simulink library "rtlsdr_book_library"  (R2018a)
settings: Solver=ode45  StartTime=0.0  StopTime=10.0  RelTol=1e-3  EnableMultiTasking=on
undefined symbols (not defined in the file): costas, den, dfilt, fdesignblkfcn, frm, gcbh, iir, num, rtlsdr_frmsize, rtlsdr_fs, src
libraries: dspsigops x6, commsynccomp2 x4, dspsrcs4 x2, dspstat3 x2, dspobslib x2, simulink_extras x2, dspmtrx3 x2, dsparch4 x1, $bdroot x1, dspspect3 x1, commrflib2 x1
(part 2 of 5)

== system rtlsdr_book_library/Additional Tools/Model Information ==
  Model Information : Subsystem
      mask help:
      | html = [html,'</br></br>',...
      |                '<table style="width:100%">',...
      |                '<tr>',...
      |                     '<td align="center" rowspan=2>',...  COL1 ROW 1
      |                         '<a href="matlab:openpdfnameddest_slxfile" STYLE="text-decoration: none">',...
      |                         '<img src="',imagepath_book,'" title="Click here to open the book at the corresponding exercise"  align="middle"/></a>',...
      |                     '</td>'];
      |         if file.videourl ~= ''''
      |             html = [html,...
      |                     '<td align="center">',...  COL 2 ROW 1
      |                         '<a href="',file.videourl,'" STYLE="text-decoration: none">',...
      |                         '<img src="',imagepath_video,'" title="Click here to watch the video"  align="middle"/></a>',...
      |                     '</td>'];
      |         end
      |         html = [html,'</tr>'];
      |
      |         if file.videourl ~= ''''
      |             html = [html,...
      |                 '<tr>',...
      |                     '<td align="center">',... COL 2 ROW 2
      |                         '<a href="',file.videourl,'" STYLE="text-decoration: none; color: #007193">',...
      |                         '<h4></br>Click here to watch the video</h4></a>',...
      |                     '</td>',...
      |                 '</tr>'];
      |         else
      |             html = [html,... ROW 2
      |                 '<tr></tr>'];
      |         end
      |         html = [html,...
      |                 '<tr>',...
      |                     '<td align="center" rowspan="2">',... COL 1 ROW 3
      |                         '<a href="matlab:openpdfnameddest_slxfile" STYLE="text-decoration: none; color: #007193">',...
      |                         '<h4></br>Click here to open the book</br>at the corresponding exercise</h4></a>',...
      |                     '</td>',...
      |                 '</tr>'];
      mask DialogControl DescGroupVar Prompt: Model Information
      mask Display:
      | % if java is installed and the help browser can be launched
      | if usejava('swing')
      | 
      |     % try to pull model properties into block
      |     try
      | 
      |         %% IMPORT FILE PARAMS
      | 
      |         % find rtlsdr book root folder
      |         root = which('rtlsdr_book_library');
      |         root = root(1:end-length('rtlsdr_book_library/rtlsdr_book_library.slx'));
      | 
      |         % find filename, path etc
      |         file.path = which(bdroot);
      |         [parentfolder,filenamenoext,fileext] = fileparts(file.path);
      |         file.relativepath = ['...',file.path(length(root):end)];
      |         file.name =[filenamenoext,fileext];
      | 
      |         % load file information cell array
      |         load('fileinfo.mat');
      | 
      |         % search to find file information
      |         row = find(ismember(fileinfo,file.name));
      | 
      |         % get remaining file information
      |         file.title = char(fileinfo(row,2));
      |         file.author = char(fileinfo(row,3));
      |         file.date = char(fileinfo(row,4));
      |         file.pdfnameddest = char(fileinfo(row,5));
      |         file.videourl = char(fileinfo(row,6));
      |         file.info1 = char(fileinfo(row,7));
      |         file.info2 = char(fileinfo(row,8));
      |         file.infoi = char(fileinfo(row,9));
      | 
      |         %% CHECK BLOCK POSITION
      |         blkpos = get_param(gcb,'Position');
      |         set_param(gcb,'Position',[blkpos(1),blkpos(2),blkpos(3),blkpos(2)+150]);
      | 
      |         %% BLOCK TEXT TITLE
      |         blktitlelen = blkpos(3)-blkpos(1)-450;
      |         blktitlecharlen = round(blktitlelen/11);
      |         blktitle = file.title;
      |         % check if title is too long to fit on one line
      |         if length(blktitle) > blktitlecharlen
      |             % find out where spaces are
      |             titlespaces = isspace(blktitle);
      |             for i = blktitlecharlen:-1:1
      |                 % if there is a space at position i
      |                 if titlespaces(i)==1
      |                     % replace with new line char
      |                     blktitle(i)=char(10);
      |                     blktitlebreakpos = i;
      |                     % break loop
      |                     break;
      |                 end
      |             end
      |         end
      |         % check if title is too long to fit on two lines
      |         if length(blktitle) > 2*blktitlecharlen
      |             % find out where spaces are
      |             titlespaces = isspace(blktitle);
      |             for i = 2*blktitlecharlen:-1:blktitlecharlen
      |                 % if there is a space at position i
      |                 if titlespaces(i)==1
      |                     % replace with new line char
      |                     blktitle(i)=char(10);
      |                     % break loop
      |                     break;
      |                 end
      |             end
      |         end
      |         % format string for mask display
      |         blkmsg = ['\bf\fontsize{20}',blktitle,'\fontsize{22}',char(10),...
      |                   '\rm\fontsize{16}www.desktopSDR.com\fontsize{18}',char(10),...
      |                   '\rm\fontsize{14}Double click for more information'];
      | 
      | 
      |         %% CREATE PARAMS FOR HTML
      |         % get MATLAB version
      |         MATLABversion = num2str(get_param(gcs,'Version'));
      |         if MATLABversion(1:3)=='8.2'
      |             file.MATLABversion = ['Last saved in Simulink version ',MATLABversion(1:3),' – R2013b'];
      |         elseif MATLABversion(1:3)=='8.3'
      |             file.MATLABversion = ['Last saved in Simulink version ',MATLABversion(1:3),' – R2014a'];
      |         elseif MATLABversion(1:3)=='8.4'
      |             file.MATLABversion = ['Last saved in Simulink version ',MATLABversion(1:3),' – R2014b'];
      |         elseif MATLABversion(1:3)=='8.5'
      |             file.MATLABversion = ['Last saved in Simulink version ',MATLABversion(1:3),' – R2015a'];
      |         elseif MATLABversion(1:3)=='8.6'
      |             file.MATLABversion = ['Last saved in Simulink version ',MATLABversion(1:3),' – R2015b'];
      |         else
      |             file.MATLABversion = ['Last saved in Simulink version ',MATLABversion(1:3)];
      |         end
      |         % image hyperlinks
      |         imagepath_book = [root,'rtlsdr_book_library/block_icons/icon__book.png'];
      |         imagepath_desktopSDR = [root,'rtlsdr_book_library/block_icons/icon__desktopSDR.png'];
      |         imagepath_video = [root,'rtlsdr_book_library/block_icons/icon__video.png'];
      | 
      | 
      |         %% CREATE HTML WEBPAGE FOR OPEN FUNCTION CALLBACK
      |         % create table at the top
      |         html = ['text://<html>',...
      |                 '<title>',bdroot,' - ',file.title,'</title>',...
      |                 '<body>',...
      |                 '<table style="width:100%" border=0 cellspacing=0 cellpadding=20">',...
      |                     '<tr>',...
      |                         '<td bgcolor="#007193" style="width: 100%;">',...
      |                         '<center><a href=http://www.desktopSDR.com>',...
      |                             '<img src="',imagepath_desktopSDR,'" title="Go to desktopSDR.com"  align="middle"/>',...
      |                         '</a></center>',...
      |                         '</td>',...
      |                     '</tr>',...
      |                 '</table></br></br>',...
      |                 '<table style="width:100%">',...
      |                     '<tr>',...
      |                         '<td class="expand"><font color="#323232" face="verdana"><h2>Model Title:</h2></td>',...
      |                         '<td><font color="#323232" face="verdana"><h2>',file.title,'</h2></td>',...
      |                     '</tr>',...
      |                     '<tr>'...
      |                         '<td class="expand"><font color="#323232" face="verdana"><h3>Model Filepath:</h3></td>',...
      |                         '<td><font color="#323232" face="verdana"><h3>',file.relativepath,'</h3></td>',...
      |                     '</tr>'...
      |                     '<tr>'...
      |                         '<td class="expand"><font color="#323232" face="verdana"><h5>Model Author:</h5></td>',...
      |                         '<td><font color="#323232" face="verdana"><h5>',file.author,'</h5></td>',...
      |                     '</tr>'...
      |                     '<tr>'...
      |                         '<td class="expand"><font color="#323232" face="verdana"><h5>Model Date:</h5></td>',...
      |                         '<td><font color="#323232" face="verdana"><h5>',file.date,'</h5></td>',...
      |                     '</tr>'...
      |                     '<tr>'...
      |                         '<td class="expand"><font color="#323232" face="verdana"><h5>Simulink Version:</h5></td>',...
      |                         '<td><font color="#323232" face="verdana"><h5>',file.MATLABversion,'</h5></td>',...
      |                     '</tr>'...
      |                     '<tr>'...
      |                         '<td><font color="#323232" face="verdana"><h5>Exercise introduction:</h5></td>',...
      |                     '</tr>'...
      |                 '</table>'];
      |         % add info paragraphs if they are populated
      |         if file.info1 ~= ''''
      |             html = [html,'<font color="#757575" face="verdana"><p align="justify">',file.info1,'</p>'];
      |         end
      |         if file.info2 ~= ''''
      |             html = [html,'<font color="#757575" face="verdana"><p align="justify">',file.info2,'</p>'];
      |         end
      |         if file.infoi ~= ''''
      |             html = [html,'<p align="justify"><i>',file.infoi,'</i></p>'];
      |         end
      |         % add hyperlinks in second table (book only if no video is provided)
      |         html = [html,'</br></br>',...
      |                '<table style="width:100%">',...
      |                '<tr>',...
      |                     '<td align="center">',...  COL 1 ROW 1
      |                         '<a href="matlab:openpdfnameddest_slxfile" STYLE="text-decoration: none">',...
      |                         '<img src="',imagepath_book,'" title="Click here to open the book at the corresponding exercise"  align="middle"/></a>',...
      |                     '</td>'];
      |         if file.videourl ~= ''''
      |             html = [html,...
      |                     '<td align="center">',...  COL 2 ROW 1
      |                         '<a href="',file.videourl,'" STYLE="text-decoration: none">',...
      |                         '<img src="',imagepath_video,'" title="Click here to watch the video"  align="middle"/></a>',...
      |                     '</td>'];
      |         end
      |         html = [html,'</tr>'];
      | 
      |         html = [html,...
      |                 '<tr>',...
      |                     '<td align="center" rowspan="2">',... COL 1 ROW 2
      |                         '<a href="matlab:openpdfnameddest_slxfile" STYLE="text-decoration: none; color: #007193">',...
      |                         '<h4></br>Click here to open the book</br>at the corresponding exercise</h4></a>',...
      |                     '</td>'];
      |         if file.videourl ~= ''''
      |             html = [html,...
      |                     '<td align="center">',... COL 2 ROW 2
      |                         '<a href="',file.videourl,'" STYLE="text-decoration: none; color: #007193">',...
      |                         '<h4></br>Click here to watch the video</h4></a>',...
      |                     '</td>',...
      |                 '</tr>'];
      |         else
      |             html = [html,... ROW 2
      |                 '</tr>'];
      |         end
      | 
      |         % finish table
      |         html = [html,'</table>'];
      | 
      |         % legal information
      |         html = [html,...
      |                 '<font color="#757575" face="verdana" size=1></br></br></br></br></br></br>',...
      |                 '</br><strong>Software, Simulation Examples and Design Exercises Licence Agreement</strong>',...
      |                 '</br><p align="justify">This license agreement refers to the simulation examples, design exercises and files, and associated software MATLAB and Simulink resources that accompany the book:',...
      |                 '</br></br>&nbsp;&nbsp;&nbsp;<em>Title: Software Defined Radio using MATLAB & Simulink and the RTL-SDR',...
      |                 '</br>&nbsp;&nbsp;&nbsp;Published by Strathclyde Academic Media, 2015',...
      |                 '</br>&nbsp;&nbsp;&nbsp;Authored by Robert W. Stewart, Kenneth W. Barlee, Dale S.W. Atkinson, and Louise H. Crockett</em>',...
      |                 '</br></br><p align="justify">and made available as a download from <a href="http://www.desktopSDR.com" STYLE="text-decoration: none">www.desktopSDR.com</a> or variously acquired by other means such as via USB storage, cloud storage, disk or any other electronic or optical or magnetic storage mechanism. These files and associated software may be used subject to the terms of agreement of the conditions below:',...
      |                 '</br></br>&nbsp;&nbsp;&nbsp;<em>Copyright © 2015 Robert W. Stewart, Kenneth W. Barlee, Dale S.W. Atkinson, and Louise H. Crockett. All rights reserved.</em>',...
      |                 '</br></br><p align="justify">Redistribution and use in source and binary forms, with or without modification, are permitted provided that the following conditions are met:',...
      |                 '<ol type="1">',...
      |                 '</br><li>Redistributions of source code must retain the above copyright notice, this list of conditions and the following disclaimer.</li>',...
      |                 '</br><li>Redistributions in binary form must reproduce the above copyright notice, this list of conditions and the following disclaimer in the documentation and/or other materials provided with the distribution.</li>',...
      |                 '</br><li>Neither the name of the copyright holder nor the names of its contributors may be used to endorse or promote products derived from this software without specific prior written permission.</li>',...
      |                 '</br><li>In all cases, the software is, and all modifications and derivatives of the software shall be, licensed to you solely for use in conjunction with The MathWorks, Inc. products and service offerings.</li>',...
      |                 '</ol>',...
      |                 '</br><p align="justify">THIS SOFTWARE IS PROVIDED BY THE COPYRIGHT HOLDERS AND CONTRIBUTORS "AS IS" AND ANY EXPRESS OR IMPLIED WARRANTIES, INCLUDING, BUT NOT LIMITED TO, THE IMPLIED WARRANTIES OF MERCHANTABILITY AND FITNESS FOR A PARTICULAR PURPOSE ARE DISCLAIMED. IN NO EVENT SHALL THE COPYRIGHT HOLDER OR CONTRIBUTORS BE LIABLE FOR ANY DIRECT, INDIRECT, INCIDENTAL, SPECIAL, EXEMPLARY, OR CONSEQUENTIAL DAMAGES (INCLUDING, BUT NOT LIMITED TO, PROCUREMENT OF SUBSTITUTE GOODS OR SERVICES; LOSS OF USE, DATA, OR PROFITS; OR BUSINESS INTERRUPTION) HOWEVER CAUSED AND ON ANY THEORY OF LIABILITY, WHETHER IN CONTRACT, STRICT LIABILITY, OR TORT (INCLUDING NEGLIGENCE OR OTHERWISE) ARISING IN ANY WAY OUT OF THE USE OF THIS SOFTWARE, EVEN IF ADVISED OF THE POSSIBILITY OF SUCH DAMAGE.</p>',...
      |                 '</br><strong>Audio Tracks used in Simulations Examples and Design Exercises</strong>',...
      |                 '<p align="justify">The music and vocal files used within the Examples files and software within the book were variously written, arranged, performed, recorded and produced by Garrey Rice, Adam Struth, Jamie Struth, Iain Thistlethwaite and also Marshall Craigmyle who collectively, and individually where appropriate, assert and retain all of their copyright, performance and artistic rights. Permission to use and reproduce this music is granted for all purposes associated with MATLAB and Simulink software and the simulation examples and design exercises files that accompany this book. Requests to use the music for any other purpose should be directed to:  info@desktopSDR.com. For information on music track names, full credits, and links to the musicians please refer to <a href="http://www.desktopSDR.com/more/audio" STYLE="text-decoration: none">www.desktopSDR.com/more/audio</a>.</p></br></br>'];
      | 
      |         % finish HTML code
      |         html = [html,...
      |                 '</font></body>',...
      |                 '</html>'];
      | 
      |         % set callback
      |         cb = ['web(''',html,''');'];
      |         set_param(gcb,'OpenFcn',eval('cb'));
      | 
      | 
      |     catch %% CANNOT LOAD PROPERTIES
      | 
      |         % format string for mask display
      |         blkmsg = 'Unable to load model information';
      |         % clear openfcn callback
      |         set_param(gcb,'OpenFcn',' ');
      | 
      |     end
      | end
      | 
      | %% DISPLAY TEXT ON BLOCK
      | text(415,75,blkmsg,'texmode','on','horizontalAlignment','left');
      | 
      | %% DISPLAY IMAGE ON BLOCK
      | try
      |     root = which('rtlsdr_book_library');
      |     root = root(1:end-length('rtlsdr_book_library/rtlsdr_book_library.slx'));
      |     imagepath = [root,'rtlsdr_book_library/block_icons/icon__booklogo.png'];
      |     image(imagepath,[0,0,400,150]);
      | end

== system rtlsdr_book_library/Additional Tools/Remove DC Component ==
  sig_in : Inport
  Mean : dspstat3/Mean  run=off  reset_popup=None  InputProcessing=Columns as channels (frame based)  directionMode=Each column  dimension=1  treatSBRowAsCol=on  roiEnable=off  roiType=Rectangles  roiPortion=Entire ROI  roiOutput=Individual statistics for each ROI  roiFlag=off  outputDataTypeStr=Inherit: Same as accumulator  outputLastDataTypeStr=Inherit: Same as accumulator  outputMin=[]  outputMax=[]  roundingMode=Floor  overflowMode=off
  Subtract : Sum  Inputs=+-
  sig_out : Outport
  wires:
  Subtract/1 -> sig_out/1
  sig_in/1 -> Subtract/1, Mean/1
  Mean/1 -> Subtract/2

== system rtlsdr_book_library/Additional Tools/Save RTL-SDR Data ==
  note: write data in 1D array to timeseries
  data_in : Inport
  Reshape : Reshape
  To File : ToFile  Filename=rtlsdr_data.mat  MatrixName=rtlsdr_data  SaveFormat=Timeseries
  wires:
  data_in/1 -> Reshape/1
  Reshape/1 -> To File/1

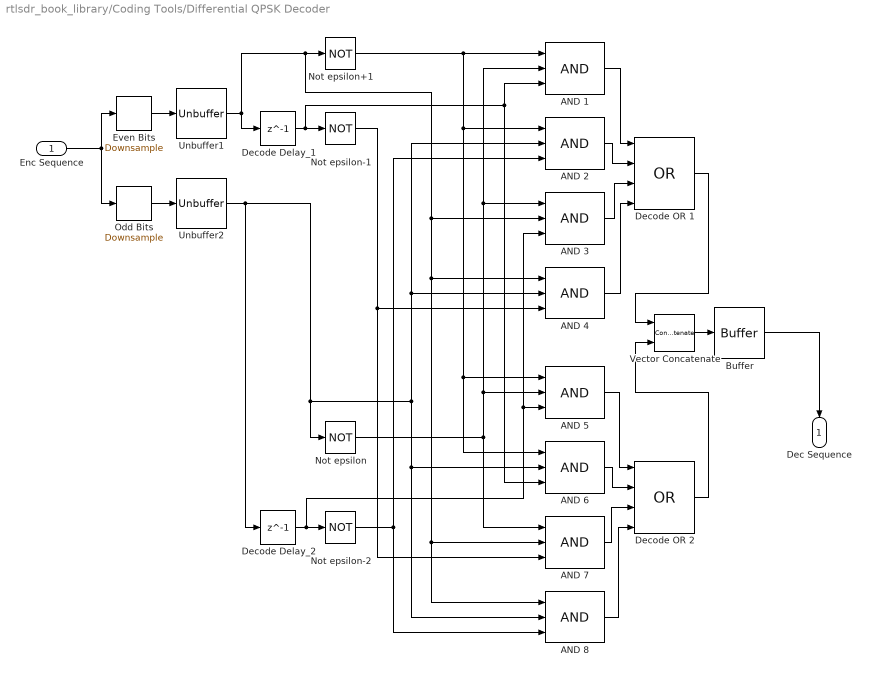
== system rtlsdr_book_library/Coding Tools/Differential QPSK Decoder ==
  Enc Sequence : Inport
  AND {1..8} (8 alike) : Logic  Inputs=3  IconShape=distinctive  AllPortsSameDT=off  OutDataTypeStr=boolean
  Buffer : Buffer  N=op_buff_len
  Decode Delay_1 : Delay  DelayLength=1  InitialCondition=0
  Decode Delay_2 : Delay  DelayLength=1  InitialCondition=0
  Decode OR 1 : Logic  Operator=OR  Inputs=4  IconShape=distinctive  AllPortsSameDT=off  OutDataTypeStr=boolean
  Decode OR 2 : Logic  Operator=OR  Inputs=4  IconShape=distinctive  AllPortsSameDT=off  OutDataTypeStr=boolean
  Even Bits : dspsigops/Downsample  N=2  phase=1  InputProcessing=Columns as channels (frame based)  RateOptions=Enforce single-rate processing  smode=Allow multirate  fmode=Maintain input frame size  ic=0
      settings: SourceProductName=DSP System Toolbox  SourceProductBaseCode=DS
  Not epsilon : Logic  Operator=NOT  Inputs=3  IconShape=distinctive  AllPortsSameDT=off  OutDataTypeStr=boolean
  Not epsilon+1 : Logic  Operator=NOT  Inputs=3  IconShape=distinctive  AllPortsSameDT=off  OutDataTypeStr=boolean
  Not epsilon-1 : Logic  Operator=NOT  Inputs=3  IconShape=distinctive  AllPortsSameDT=off  OutDataTypeStr=boolean
  Not epsilon-2 : Logic  Operator=NOT  Inputs=3  IconShape=distinctive  AllPortsSameDT=off  OutDataTypeStr=boolean
  Odd Bits : dspsigops/Downsample  N=2  phase=0  InputProcessing=Columns as channels (frame based)  RateOptions=Enforce single-rate processing  smode=Allow multirate  fmode=Maintain input frame size  ic=0
      settings: SourceProductName=DSP System Toolbox  SourceProductBaseCode=DS
  Unbuffer1 : Unbuffer
  Unbuffer2 : Unbuffer
  Vector Concatenate : Concatenate
  Dec Sequence : Outport
  wires:
  Not epsilon-2/1 -> AND 2/3, AND 8/3
  Decode OR 2/1 -> Vector Concatenate/2
  Decode Delay_2/1 -> Not epsilon-2/1, AND 3/3, AND 5/3
  Unbuffer1/1 -> Not epsilon+1/1, AND 7/2, AND 8/1, AND 4/1, AND 3/2, Decode Delay_1/1
  Buffer/1 -> Dec Sequence/1
  AND 5/1 -> Decode OR 2/1
  AND 2/1 -> Decode OR 1/2
  Enc Sequence/1 -> Odd Bits/1, Even Bits/1
  AND 3/1 -> Decode OR 1/3
  AND 7/1 -> Decode OR 2/3
  Not epsilon+1/1 -> AND 1/1, AND 6/1, AND 5/1, AND 2/1
  AND 6/1 -> Decode OR 2/2
  Not epsilon/1 -> AND 3/1, AND 1/2, AND 5/2, AND 7/1
  AND 1/1 -> Decode OR 1/1
  AND 4/1 -> Decode OR 1/4
  Even Bits/1 -> Unbuffer1/1
  Odd Bits/1 -> Unbuffer2/1
  Decode OR 1/1 -> Vector Concatenate/1
  Not epsilon-1/1 -> AND 7/3, AND 4/3
  Unbuffer2/1 -> Not epsilon/1, AND 2/2, AND 4/2, AND 6/2, AND 8/2, Decode Delay_2/1
  Decode Delay_1/1 -> Not epsilon-1/1, AND 1/3, AND 6/3
  AND 8/1 -> Decode OR 2/4
  Vector Concatenate/1 -> Buffer/1

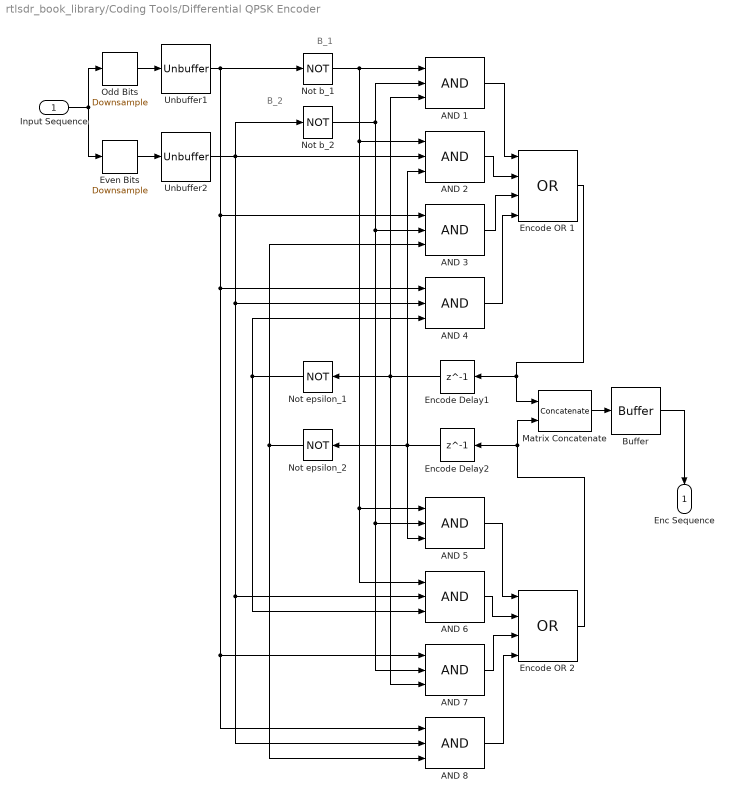
== system rtlsdr_book_library/Coding Tools/Differential QPSK Encoder ==
  note: B_2
  note: B_1
  Input Sequence : Inport
  AND {1..8} (8 alike) : Logic  Inputs=3  IconShape=distinctive  AllPortsSameDT=off  OutDataTypeStr=boolean
  Buffer : Buffer  N=op_buff_len
  Encode Delay1 : Delay  DelayLength=1  InitialCondition=0
  Encode Delay2 : Delay  DelayLength=1  InitialCondition=0
  Encode OR 1 : Logic  Operator=OR  Inputs=4  IconShape=distinctive  AllPortsSameDT=off  OutDataTypeStr=boolean
  Encode OR 2 : Logic  Operator=OR  Inputs=4  IconShape=distinctive  AllPortsSameDT=off  OutDataTypeStr=boolean
  Even Bits : dspsigops/Downsample  N=2  phase=1  InputProcessing=Columns as channels (frame based)  RateOptions=Enforce single-rate processing  smode=Allow multirate  fmode=Maintain input frame size  ic=0
      settings: SourceProductName=DSP System Toolbox  SourceProductBaseCode=DS
  Matrix Concatenate : Concatenate  ConcatenateDimension=2
  Not b_1 : Logic  Operator=NOT  Inputs=3  IconShape=distinctive  AllPortsSameDT=off  OutDataTypeStr=boolean
  Not b_2 : Logic  Operator=NOT  Inputs=3  IconShape=distinctive  AllPortsSameDT=off  OutDataTypeStr=boolean
  Not epsilon_1 : Logic  Operator=NOT  Inputs=3  IconShape=distinctive  AllPortsSameDT=off  OutDataTypeStr=boolean
  Not epsilon_2 : Logic  Operator=NOT  Inputs=3  IconShape=distinctive  AllPortsSameDT=off  OutDataTypeStr=boolean
  Odd Bits : dspsigops/Downsample  N=2  phase=0  InputProcessing=Columns as channels (frame based)  RateOptions=Enforce single-rate processing  smode=Allow multirate  fmode=Maintain input frame size  ic=0
      settings: SourceProductName=DSP System Toolbox  SourceProductBaseCode=DS
  Unbuffer1 : Unbuffer
  Unbuffer2 : Unbuffer
  Enc Sequence : Outport
  wires:
  Encode Delay1/1 -> Not epsilon_1/1, AND 1/3, AND 7/3
  Encode Delay2/1 -> Not epsilon_2/1, AND 5/3, AND 2/3
  Not epsilon_2/1 -> AND 8/3, AND 3/3
  AND 1/1 -> Encode OR 1/1
  AND 8/1 -> Encode OR 2/4
  Even Bits/1 -> Unbuffer2/1
  Input Sequence/1 -> Even Bits/1, Odd Bits/1
  Odd Bits/1 -> Unbuffer1/1
  Encode OR 2/1 -> Matrix Concatenate/2, Encode Delay2/1
  Encode OR 1/1 -> Matrix Concatenate/1, Encode Delay1/1
  AND 2/1 -> Encode OR 1/2
  Not b_2/1 -> AND 7/2, AND 5/2, AND 3/2, AND 1/2
  Unbuffer1/1 -> Not b_1/1, AND 3/1, AND 4/1, AND 7/1, AND 8/1
  AND 6/1 -> Encode OR 2/2
  AND 7/1 -> Encode OR 2/3
  AND 5/1 -> Encode OR 2/1
  Not epsilon_1/1 -> AND 6/3, AND 4/3
  AND 4/1 -> Encode OR 1/4
  Not b_1/1 -> AND 1/1, AND 6/1, AND 5/1, AND 2/1
  AND 3/1 -> Encode OR 1/3
  Unbuffer2/1 -> AND 2/2, AND 4/2, AND 6/2, AND 8/2, Not b_2/1
  Matrix Concatenate/1 -> Buffer/1
  Buffer/1 -> Enc Sequence/1

== system rtlsdr_book_library/Data Comms Sources and Sinks/  ASCII Transfer Binary Source ==
  MATLAB Function : MATLAB Function  TreatAsAtomicUnit=on
  Obtain Frame (header & data) : Constant  Value=src.master_frame  VectorParams1D=off  SampleTime=1/src.fs*(length(src.master_frame))
  Obtain count_lim : Constant  Value=src.count_lim  VectorParams1D=off  SampleTime=1/src.fs*(length(src.master_frame))
  data_out : Outport
  wires:
  Obtain count_lim/1 -> MATLAB Function/1(count_lim)
  Obtain Frame (header & data)/1 -> MATLAB Function/2(master_frame)
  MATLAB Function/1(frame_output) -> data_out/1

== system rtlsdr_book_library/Data Comms Sources and Sinks/ASCII Decoding ==
  frame_payload_in : Inport
  Ascii Length : Constant  Value=ascii_len  VectorParams1D=off  OutDataTypeStr=single  FramePeriod=4096/240e3
  Binary to ASCII : MATLAB Function  TreatAsAtomicUnit=on
      mask init:
      | %% FIGURE SETUP        
      | %figure;
      | 
      | % resize
      | %window_x = 500;
      | %window_y = 500;
      | %window_width = 500;
      | %window_height = 110;
      | %set(gcf, 'Position', [window_x window_y window_width window_height]);
      | %set(gcf, 'menubar', 'none');
  Message Length : Constant  Value=msg_len  VectorParams1D=off  OutDataTypeStr=single  FramePeriod=-1
  wires:
  Message Length/1 -> Binary to ASCII/2(msg_len)
  Ascii Length/1 -> Binary to ASCII/3(ascii_len)
  frame_payload_in/1 -> Binary to ASCII/1(msg)

== system rtlsdr_book_library/Data Comms Sources and Sinks/Image Reconstruction ==
  frame_in : Inport
  Binary Length of Pixel : Constant  Value=frm.binary_len  VectorParams1D=off  OutDataTypeStr=single  FramePeriod=-1
  Image Reconstruction : MATLAB Function  TreatAsAtomicUnit=on
  wires:
  frame_in/1 -> Image Reconstruction/1(frame_in)
  Binary Length of Pixel/1 -> Image Reconstruction/2(binary_len)

== system rtlsdr_book_library/Data Comms Sources and Sinks/Image Transfer Binary Source ==
  MATLAB Function : MATLAB Function  TreatAsAtomicUnit=on
  Obtain Frame (header & data) : Constant  Value=frm.master_frame  VectorParams1D=off  SampleTime=1/frm.fs*(frm.frame_len)
  Obtain number of frames : Constant  Value=frm.no_of_frames  VectorParams1D=off  SampleTime=1/frm.fs*(frm.frame_len)
  data_out : Outport
  wires:
  Obtain number of frames/1 -> MATLAB Function/1(count_lim)
  Obtain Frame (header & data)/1 -> MATLAB Function/2(master_frame)
  MATLAB Function/1(frame_output) -> data_out/1

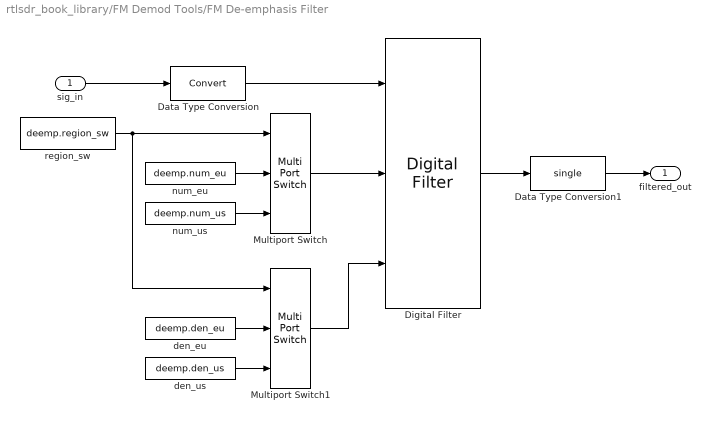
== system rtlsdr_book_library/FM Demod Tools/FM De-emphasis Filter ==
  sig_in : Inport
  Data Type Conversion : DataTypeConversion
  Data Type Conversion1 : DataTypeConversion  OutDataTypeStr=single
  Digital Filter : dspobslib/Digital Filter  TypePopup=IIR (poles & zeros)  IIRFiltStruct=Direct form I  AllPoleFiltStruct=Direct form  FIRFiltStruct=Direct form  CoeffSource=Input port(s)  NumCoeffs=[1 2]  DenCoeffs=[1 0.1]  BiQuadCoeffs=[1 0.3 0.4 1 0.1 0.2]  LatticeCoeffs=[0.2 0.4]  denIgnore=off  FiltPerSampPopup=One filter per frame  IC=0  ICnum=0  ICden=0  roundingMode=Floor  overflowMode=off  ScaleValues=1  scaleValueFracLength=14  stageInFracLength=15  stageOutFracLength=15  FilterSource=Input port(s)  dfiltObjectName=dfilt.df1(num,den)  InputProcessing=Columns as channels (frame based)
      settings: SourceProductName=DSP System Toolbox  SourceProductBaseCode=DS
  Multiport Switch : MultiPortSwitch  Inputs=2
  Multiport Switch1 : MultiPortSwitch  Inputs=2
  den_eu : Constant  Value=deemp.den_eu
  den_us : Constant  Value=deemp.den_us
  num_eu : Constant  Value=deemp.num_eu
  num_us : Constant  Value=deemp.num_us
  region_sw : Constant  Value=deemp.region_sw
  filtered_out : Outport
  wires:
  Multiport Switch1/1 -> Digital Filter/3
  Multiport Switch/1 -> Digital Filter/2
  den_us/1 -> Multiport Switch1/3
  den_eu/1 -> Multiport Switch1/2
  region_sw/1 -> Multiport Switch/1, Multiport Switch1/1
  num_us/1 -> Multiport Switch/3
  num_eu/1 -> Multiport Switch/2
  Digital Filter/1 -> Data Type Conversion1/1
  sig_in/1 -> Data Type Conversion/1
  Data Type Conversion/1 -> Digital Filter/1
  Data Type Conversion1/1 -> filtered_out/1

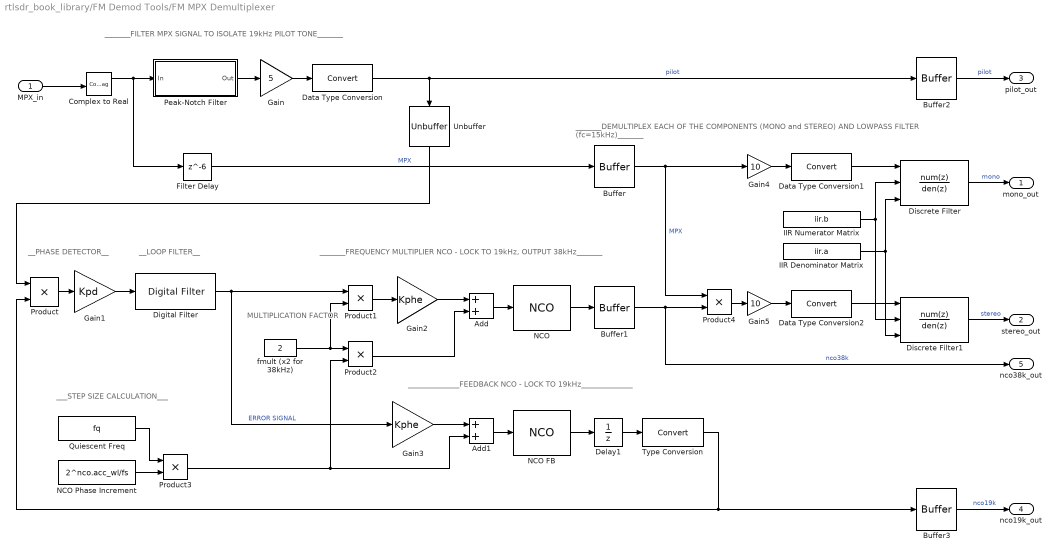
== system rtlsdr_book_library/FM Demod Tools/FM MPX Demultiplexer ==
  note: ______________FEEDBACK NCO - LOCK TO 19kHz______________
  note: _______FREQUENCY MULTIPLIER NCO - LOCK TO 19kHz, OUTPUT 38kHz_______
  note: __PHASE DETECTOR__
  note: __LOOP FILTER__
  note: ___STEP SIZE CALCULATION___
  note: MULTIPLICATION
      | FACTOR
  note: _______DEMULTIPLEX EACH OF THE COMPONENTS (MONO and STEREO) AND LOWPASS FILTER (fc=15kHz)_______
  note: _______FILTER MPX SIGNAL TO ISOLATE 19kHz PILOT TONE_______
  MPX_in : Inport
  Add : Sum  InputSameDT=on  OutDataTypeStr=Inherit: Same as first input
  Add1 : Sum  InputSameDT=on  OutDataTypeStr=Inherit: Same as first input
  Buffer{,1..3} (4 alike) : Buffer  N=frm_size
  Complex to Real : ComplexToRealImag
  Data Type Conversion : DataTypeConversion
  Data Type Conversion1 : DataTypeConversion
  Data Type Conversion2 : DataTypeConversion
  Delay1 : UnitDelay  SampleTime=1/fs
  Digital Filter : dspobslib/Digital Filter  TypePopup=IIR (poles & zeros)  IIRFiltStruct=Direct form II transposed  AllPoleFiltStruct=Direct form  FIRFiltStruct=Direct form  CoeffSource=Specify via dialog  NumCoeffs=[0,1,-0.994711805058698]  DenCoeffs=[1,-1.96959417190845,0.969594171908450]  BiQuadCoeffs=[1 0.3 0.4 1 0.1 0.2]  LatticeCoeffs=[0.2 0.4]  denIgnore=on  FiltPerSampPopup=One filter per frame  IC=0  ICnum=0  ICden=0  roundingMode=Nearest  overflowMode=off  ScaleValues=1  scaleValueFracLength=14  stageInFracLength=15  stageOutFracLength=15  FilterSource=Specify via dialog  dfiltObjectName=dfilt.dffir([1 2 1])  InputProcessing=Inherited (this choice will be removed - see release notes)
      settings: SourceProductName=DSP System Toolbox  SourceProductBaseCode=DS
  Discrete Filter : DiscreteFilter  NumeratorSource=Input port  Numerator=[0.5 0.5]  DenominatorSource=Input port  Denominator=[1 0.1]  InputProcessing=Columns as channels (frame based)  FilterStructure=Direct form II transposed  a0EqualsOne=on
      settings: InputPortMap=u0,p1,p3
  Discrete Filter1 : DiscreteFilter  NumeratorSource=Input port  Numerator=[0.5 0.5]  DenominatorSource=Input port  Denominator=[1 0.1]  InputProcessing=Columns as channels (frame based)  FilterStructure=Direct form II transposed  a0EqualsOne=on
      settings: InputPortMap=u0,p1,p3
  Filter Delay : Delay  DelayLength=6  InputProcessing=Columns as channels (frame based)
  Gain : Gain  Gain=5
  Gain1 : Gain  Gain=Kpd  OutDataTypeStr=double
  Gain2 : Gain  Gain=Kphe  OutDataTypeStr=uint32
  Gain3 : Gain  Gain=Kphe  OutDataTypeStr=uint32
  Gain4 : Gain  Gain=10
  Gain5 : Gain  Gain=10
  IIR Denominator Matrix : Constant  Value=iir.a
  "IIR Numerator Matrix " : Constant  Value=iir.b
  NCO : dspsigops/NCO  AccIncSrc=Input port  AccInc=100  PhaseOffsetSrc=Specify via dialog  PhaseOffset=0  AccumWL=nco.acc_wl  HasDither=on  DitherWL=nco.dither  PNgeneratorLength=19  HasPhaseQuantizer=on  TableDepth=nco.acc_quant  HasOutputPhaseError=off  Formula=Cosine  DataType=Binary point scaling  OutputWL=nco.op_wl  OutputFL=nco.op_frac  CompMethod=Table lookup (no interpolation)  SampleTime=1  SamplesPerFrame=1
      settings: SourceProductName=DSP System Toolbox  SourceProductBaseCode=DS
  NCO FB : dspsigops/NCO  AccIncSrc=Input port  AccInc=100  PhaseOffsetSrc=Specify via dialog  PhaseOffset=0  AccumWL=nco.acc_wl  HasDither=on  DitherWL=nco.dither  PNgeneratorLength=19  HasPhaseQuantizer=on  TableDepth=nco.acc_quant  HasOutputPhaseError=off  Formula=Cosine  DataType=Binary point scaling  OutputWL=nco.op_wl  OutputFL=nco.op_frac  CompMethod=Table lookup (no interpolation)  SampleTime=1  SamplesPerFrame=1
      settings: SourceProductName=DSP System Toolbox  SourceProductBaseCode=DS
  NCO Phase Increment : Constant  Value=2^nco.acc_wl/fs  OutDataTypeStr=uint32
  Peak-Notch Filter : Subsystem  DialogController=fdesignblkfcn  mask(Peak/Notch Filter){}
      mask help: Design a peak/notch filter
      mask Help: helpview(mapfilelocation('dsp'), 'dsppeaknotchfilter');
      mask Display: disp('Peak-Notch');
  Product : Product
  Product1 : Product  OutDataTypeStr=uint32
  Product2 : Product  OutDataTypeStr=uint32
  Product3 : Product  OutDataTypeStr=uint32
  Product4 : Product
  Quiescent Freq : Constant  Value=fq  OutDataTypeStr=uint32
  Type Conversion : DataTypeConversion
  "Unbuffer  " : Unbuffer
  fmult (x2 for 38kHz) : Constant  Value=2
  mono_out : Outport
  stereo_out : Outport  Port=2
  pilot_out : Outport  Port=3
  nco19k_out : Outport  Port=4
  nco38k_out : Outport  Port=5
  wires:
  Product1/1 -> Gain2/1
  Add/1 -> NCO/1
  Product2/1 -> Add/2
  Gain2/1 -> Add/1
  NCO Phase Increment/1 -> Product3/2
  Quiescent Freq/1 -> Product3/1
  Gain3/1 -> Add1/1
  Add1/1 -> NCO FB/1
  NCO FB/1 -> Delay1/1
  Delay1/1 -> Type Conversion/1
  Type Conversion/1 -> Buffer3/1, Product/2
  Gain1/1 -> Digital Filter/1
  Product/1 -> Gain1/1
  "Unbuffer  "/1 -> Product/1
  fmult (x2 for 38kHz)/1 -> Product1/2, Product2/1
  Product3/1 -> Add1/2, Product2/2
  Digital Filter/1 -> Gain3/1, Product1/1  "ERROR SIGNAL"
  Gain/1 -> Data Type Conversion/1
  NCO/1 -> Buffer1/1
  Buffer1/1 -> Product4/2, nco38k_out/1  "nco38k"
  Buffer/1 -> Gain4/1, Product4/1  "MPX"
  Product4/1 -> Gain5/1
  Gain4/1 -> Data Type Conversion1/1
  MPX_in/1 -> Complex to Real/1
  Complex to Real/1 -> Peak-Notch Filter/1(In), Filter Delay/1
  Discrete Filter/1 -> mono_out/1  "mono"
  Gain5/1 -> Data Type Conversion2/1
  Discrete Filter1/1 -> stereo_out/1  "stereo"
  "IIR Numerator Matrix "/1 -> Discrete Filter1/2, Discrete Filter/2
  IIR Denominator Matrix/1 -> Discrete Filter1/3, Discrete Filter/3
  Data Type Conversion1/1 -> Discrete Filter/1
  Data Type Conversion2/1 -> Discrete Filter1/1
  Peak-Notch Filter/1(Out) -> Gain/1
  Filter Delay/1 -> Buffer/1  "MPX"
  Buffer2/1 -> pilot_out/1  "pilot"
  Buffer3/1 -> nco19k_out/1  "nco19k"
  Data Type Conversion/1 -> Buffer2/1, "Unbuffer  "/1  "pilot"

== system rtlsdr_book_library/FM Demod Tools/FM Tuner Freq and Gain Control ==
  Constant1 : Constant
  Freq : Gain  Gain=tuner_freq
  Gain : Gain  Gain=tuner_gain
  MHz : Constant  Value=1e6
  freq_out : Outport
  gain_out : Outport  Port=2
  wires:
  Freq/1 -> freq_out/1
  Gain/1 -> gain_out/1
  MHz/1 -> Freq/1
  Constant1/1 -> Gain/1

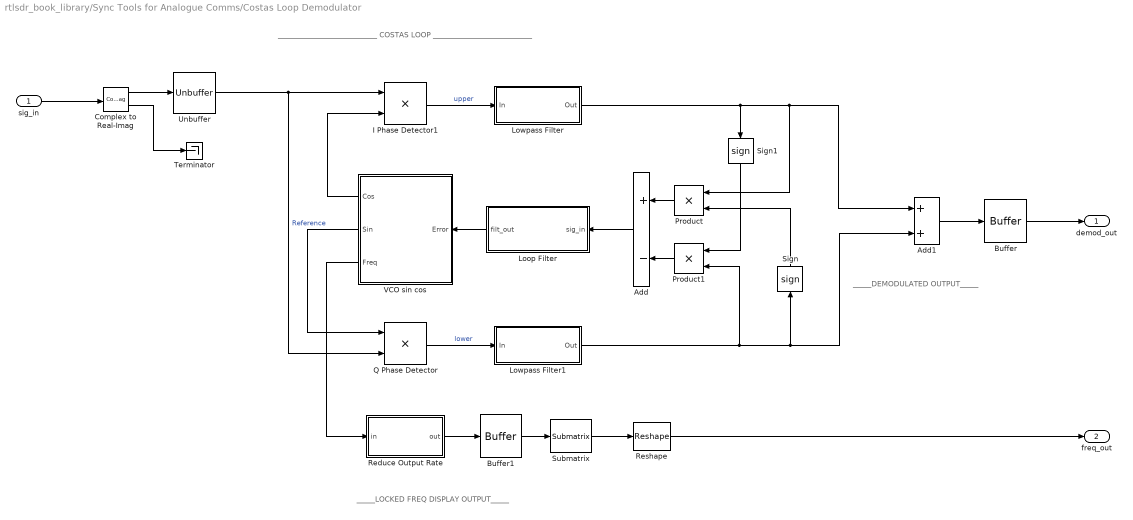
== system rtlsdr_book_library/Sync Tools for Analogue Comms/Costas Loop Demodulator ==
  note: ___________________________ COSTAS LOOP ___________________________
  note: _____DEMODULATED OUTPUT_____
  note: _____LOCKED FREQ DISPLAY OUTPUT_____
  sig_in : Inport
  Add : Sum  Inputs=+-
  Add1 : Sum  SampleTime=1/fs
  Buffer : Buffer  N=frm_size
  Buffer1 : Buffer  N=frm_size
  Complex to Real-Imag : ComplexToRealImag
  I Phase Detector1 : Product  OutDataTypeStr=single
  Loop Filter : Subsystem  mask(Loop Filter){K1=costas.K1, K2=costas.K2}
      mask prompts: K1 "K1 (proportional path) :"; K2 "K2 (integral path) :"
      mask help: This loop filter contains two paths: a proportional path with scaling coefficient K1, and an integral path with scaling coefficient K2.
      mask DialogControl Container2 Prompt: Parameters
  Lowpass Filter : Subsystem  DialogController=fdesignblkfcn  InitFcn=fdesignblkfcn(gcbh, {'InitFcn'});  mask(Lowpass Filter){}
      mask help: Design a lowpass filter
      mask Help: helpview(mapfilelocation('dsp'), 'dsplowpassfilter');
      mask Display: disp('Lowpass')
  Lowpass Filter1 : Subsystem  DialogController=fdesignblkfcn  InitFcn=fdesignblkfcn(gcbh, {'InitFcn'});  mask(Lowpass Filter){}
      mask help: Design a lowpass filter
      mask Help: helpview(mapfilelocation('dsp'), 'dsplowpassfilter');
      mask Display: disp('Lowpass')
  Product : Product
  Product1 : Product
  Q Phase Detector : Product  OutDataTypeStr=single
  Reduce Output Rate : Subsystem  mask{rate=10, fs=fs}
      mask prompts: rate "Output Rate (Hz):"; fs "System Sampling Rate (Hz):"
      mask help: Reduce the sampling rate of a signal (keep every n-th frame)
  Reshape : Reshape
  Sign : Signum
  Sign1 : Signum
  Submatrix : dspmtrx3/Submatrix  RowSpan=One row  RowStartMode=First  RowStartIndex=1  RowEndMode=Last  RowEndIndex=1  ColSpan=One column  ColStartMode=First  ColStartIndex=1  ColEndMode=Last  ColEndIndex=1
  Terminator : Terminator
  Unbuffer : Unbuffer
  VCO sin cos : Subsystem  mask(Quadratude VCO){fq=fq, sensitivity=Ko*fs}
      mask prompts: fq "Quiescent Frequency (Hz)"; sensitivity "Sensitivity (Hz/V)"
      mask help: This VCO provides both cosine and sine outputs. The quiescent frequency and sensitivity of the VCO can be defined via the mask (and these apply to both sine and cosine outputs). The block also provides the instantaneous frequency as an output.
  demod_out : Outport
  freq_out : Outport  Port=2
  wires:
  Reshape/1 -> freq_out/1
  Lowpass Filter/1(Out) -> Product/1, Add1/1, Sign1/1
  Product1/1 -> Add/2
  VCO sin cos/1(Cos) -> I Phase Detector1/2
  Reduce Output Rate/1(out) -> Buffer1/1
  Sign/1 -> Product/2
  Sign1/1 -> Product1/1
  sig_in/1 -> Complex to Real-Imag/1
  Submatrix/1 -> Reshape/1
  I Phase Detector1/1 -> Lowpass Filter/1(In)  "upper"
  Buffer1/1 -> Submatrix/1
  VCO sin cos/2(Sin) -> Q Phase Detector/1
  Add1/1 -> Buffer/1
  Q Phase Detector/1 -> Lowpass Filter1/1(In)  "lower"
  Product/1 -> Add/1
  Lowpass Filter1/1(Out) -> Add1/2, Sign/1, Product1/2
  Complex to Real-Imag/1 -> Unbuffer/1
  Complex to Real-Imag/2 -> Terminator/1
  Buffer/1 -> demod_out/1
  Unbuffer/1 -> Q Phase Detector/2, I Phase Detector1/1  "Reference"
  VCO sin cos/3(Freq) -> Reduce Output Rate/1(in)
  Loop Filter/1(filt_out) -> VCO sin cos/1(Error)
  Add/1 -> Loop Filter/1(sig_in)

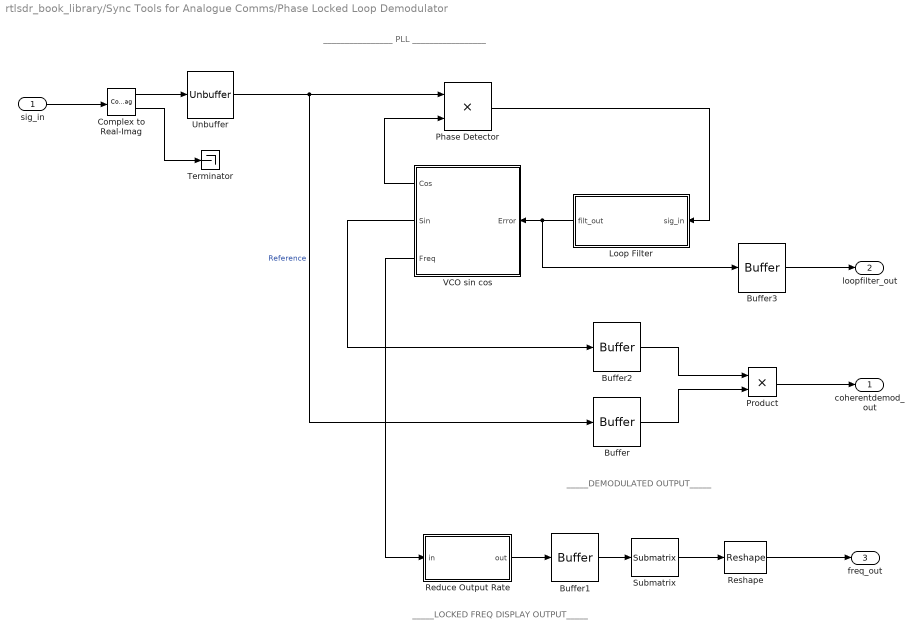
== system rtlsdr_book_library/Sync Tools for Analogue Comms/Phase Locked Loop Demodulator ==
  note: ________________ PLL _________________
  note: _____DEMODULATED OUTPUT_____
  note: _____LOCKED FREQ DISPLAY OUTPUT_____
  sig_in : Inport
  Buffer{,1..3} (4 alike) : Buffer  N=frm_size
  Complex to Real-Imag : ComplexToRealImag
  Loop Filter : Subsystem  mask(Loop Filter){K1=pll.K1, K2=pll.K2}
      mask prompts: K1 "K1 (proportional path) :"; K2 "K2 (integral path) :"
      mask help: This loop filter contains two paths: a proportional path with scaling coefficient K1, and an integral path with scaling coefficient K2.
      mask DialogControl Container2 Prompt: Parameters
  Phase Detector : Product
  Product : Product
  Reduce Output Rate : Subsystem  mask{rate=10, fs=fs}
      mask prompts: rate "Output Rate (Hz):"; fs "System Sampling Rate (Hz):"
      mask help: Reduce the sampling rate of signal (keep only every n-th frame)
  Reshape : Reshape
  Submatrix : dspmtrx3/Submatrix  RowSpan=One row  RowStartMode=First  RowStartIndex=1  RowEndMode=Last  RowEndIndex=1  ColSpan=One column  ColStartMode=First  ColStartIndex=1  ColEndMode=Last  ColEndIndex=1
  Terminator : Terminator
  Unbuffer : Unbuffer
  VCO sin cos : Subsystem  mask(Quadratude VCO){fq=fq, sensitivity=Ko*fs}
      mask prompts: fq "Quiescent Frequency (Hz)"; sensitivity "Sensitivity (Hz/V)"
      mask help: This VCO provides both cosine and sine outputs. The quiescent frequency and sensitivity of the VCO can be defined via the mask (and these apply to both sine and cosine outputs). The block also provides the instantaneous frequency as an output.
  coherentdemod_out : Outport
  loopfilter_out : Outport  Port=2
  freq_out : Outport  Port=3
  wires:
  sig_in/1 -> Complex to Real-Imag/1
  Unbuffer/1 -> Phase Detector/1, Buffer/1  "Reference"
  VCO sin cos/1(Cos) -> Phase Detector/2
  Phase Detector/1 -> Loop Filter/1(sig_in)
  VCO sin cos/2(Sin) -> Buffer2/1
  Buffer2/1 -> Product/1
  Product/1 -> coherentdemod_out/1
  Buffer/1 -> Product/2
  Loop Filter/1(filt_out) -> Buffer3/1, VCO sin cos/1(Error)
  Reduce Output Rate/1(out) -> Buffer1/1
  Buffer1/1 -> Submatrix/1
  VCO sin cos/3(Freq) -> Reduce Output Rate/1(in)
  Submatrix/1 -> Reshape/1
  Reshape/1 -> freq_out/1
  Complex to Real-Imag/1 -> Unbuffer/1
  Complex to Real-Imag/2 -> Terminator/1
  Buffer3/1 -> loopfilter_out/1

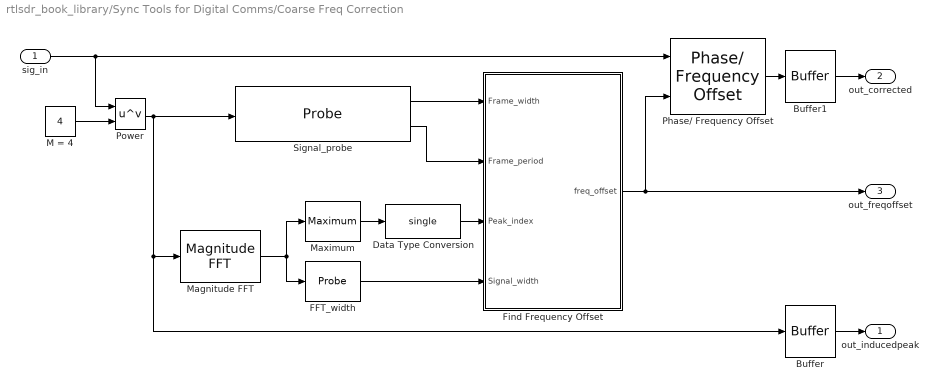
== system rtlsdr_book_library/Sync Tools for Digital Comms/Coarse Freq Correction ==
  sig_in : Inport
  Buffer : Buffer  N=frm_size
  Buffer1 : Buffer  N=frm_size
  Data Type Conversion : DataTypeConversion  OutDataTypeStr=single
  FFT_width : Probe  ProbeSampleTime=off  ProbeComplexSignal=off  ProbeWidthDataType=single  ProbeSampleTimeDataType=single
  Find Frequency Offset : MATLAB Function  TreatAsAtomicUnit=on
  M = 4 : Constant  Value=4  OutDataTypeStr=single
  Magnitude FFT : dspspect3/Magnitude FFT  mag_or_magsq=Magnitude squared  FFTImplementation=Auto  fftLenInherit=on  fftsize=1024  WrapInput=on
      settings: SourceProductName=DSP System Toolbox  SourceProductBaseCode=DS
  Maximum : dspstat3/Maximum  fcn=Index  reset=None  InputProcessing=Columns as channels (frame based)  indexBase=One  operateOver=Each column  Dimension=1  colComp=on  operation=maximum  roiEnable=off  roiType=Rectangles  roiPortion=Entire ROI  roiOutput=Individual statistics for each ROI  roiFlag=off  accumDataTypeStr=Inherit: Same as product output  accumLastDataTypeStr=Inherit: Same as product output  roundingMode=Floor  overflowMode=off
  Phase/ Frequency Offset : commrflib2/Phase// Frequency Offset  phaseOffset=0  freqPort=on  freqOffset=0
      settings: SourceProductName=Communications System Toolbox
  Power : Math  Operator=pow  OutputSignalType=complex  SaturateOnIntegerOverflow=on
  Signal_probe : Probe  ProbeComplexSignal=off  ProbeWidthDataType=single  ProbeSampleTimeDataType=single
  out_inducedpeak : Outport
  out_corrected : Outport  Port=2
  out_freqoffset : Outport  Port=3
  wires:
  Power/1 -> Signal_probe/1, Magnitude FFT/1, Buffer/1
  Signal_probe/2 -> Find Frequency Offset/2(Frame_period)
  FFT_width/1 -> Find Frequency Offset/4(Signal_width)
  M = 4/1 -> Power/2
  Signal_probe/1 -> Find Frequency Offset/1(Frame_width)
  Magnitude FFT/1 -> Maximum/1, FFT_width/1
  sig_in/1 -> Power/1, Phase/ Frequency Offset/1
  Phase/ Frequency Offset/1 -> Buffer1/1
  Maximum/1 -> Data Type Conversion/1
  Data Type Conversion/1 -> Find Frequency Offset/3(Peak_index)
  Find Frequency Offset/1(freq_offset) -> out_freqoffset/1, Phase/ Frequency Offset/2
  Buffer1/1 -> out_corrected/1
  Buffer/1 -> out_inducedpeak/1

== system rtlsdr_book_library/Additional Tools/AM-SSB Modulator/Hilbert Filter ==
  In : Inport
  Generated Filter Block : Subsystem  Tag=FilterWizardSubSystem
      settings: ErrorFcn=dspFilterRealizedInBasicElemsAlgLoopErrFcnCallback
  Out : Outport
  wires:
  Generated Filter Block/1(Output) -> Out/1
  In/1 -> Generated Filter Block/1(Input)

== system rtlsdr_book_library/Additional Tools/Model Information/Model Information ==
  Constant : Constant
  Terminator : Terminator
  wires:
  Constant/1 -> Terminator/1

== system rtlsdr_book_library/FM Demod Tools/FM MPX Demultiplexer/Peak-Notch Filter ==
  In : Inport
  Generated Filter Block : dsparch4/Biquad Filter  Tag=BlockMethodSubSystem  IIRFiltStruct=Direct form II  CoeffSource=Specify via dialog  BiQuadCoeffs=[0.0083392806558967407 -0.016678561311793474 0.0083392806558967355 1 -1.0916485720976647 0.99738928062166954;0.0030175126661685031 0 -0.0030175126661685031 1 -1.0840484113399906 0.99738159148297845;0.32375855758621658 0.64751711517243304 0.32375855758621636 1 -1.0864337865299356 0.9947776723347781]  a0Flag=Warning  IC=0  ICnum=0  ICden=0  InputProcessing=Columns as channels (frame based)  denAccumFracLength=30  denProdOutputFracLength=30  secondMemoryFracLength=15  roundingMode=Floor  overflowMode=off  ScaleValues=[0.002190967548082783;1;1;1]  optimizeScaleValues=off  ScaleValueMode=Specify via input port (g)  scaleValueFracLength=14  FilterSource=Specify via dialog  dfiltObjectName=dfilt.df2tsos([1 0.3 0.4],[1 0.1 0.2])
      settings: SourceProductName=DSP System Toolbox
  Out : Outport
  wires:
  Generated Filter Block/1 -> Out/1
  In/1 -> Generated Filter Block/1

== system rtlsdr_book_library/Sync Tools for Analogue Comms/Costas Loop Demodulator/Loop Filter ==
  note: _______INTEGRAL PATH_______
  note: _____PROPORTIONAL PATH_____
  sig_in : Inport
  Add : Sum
  Add1 : Sum  AccumDataTypeStr=single  OutDataTypeStr=single
  Delay : Delay  DelayLength=1  InitialCondition=0.00
  Gain1 : Gain  Gain=K2  OutDataTypeStr=single
  Gain2 : Gain  Gain=K1  ParamDataTypeStr=single
  filt_out : Outport
  wires:
  Gain1/1 -> Add/1
  Gain2/1 -> Add1/1
  sig_in/1 -> Gain1/1, Gain2/1
  Add/1 -> Add1/2, Delay/1
  Delay/1 -> Add/2
  Add1/1 -> filt_out/1

== system rtlsdr_book_library/Sync Tools for Analogue Comms/Costas Loop Demodulator/Lowpass Filter ==
  In : Inport
  Generated Filter Block : DiscreteFir  Tag=BlockMethodSubSystem  Coefficients=[0.0011881646839486063 0.0018650557342877545 0.0024432362147616925 0.0021354822806999088 0.00042299683017990954 -0.002811975217901171 -0.0070281841500527019 -0.010990641854786024 -0.013057295684674336 -0.011759378475939258 -0.0065122691275265243 0.0018310718678320899 0.010886986001758246 0.017273021293018758 0.017716569217906979 0.010432097914051745 -0.0037412800759900403 -0.020924513549760219 -0.03484310128301845 -0.038475584236764698 -0.026293991768716812 0.003623882030617088 0.048364704584590926 0.10035872397535391 0.14905800205298941 0.18368133717457233 0.19620901660625717 0.18368133717457233 0.14905800205298941 0.10035872397535391 0.048364704584590926 0.003623882030617088 -0.026293991768716812 -0.038475584236764698 -0.03484310128301845 -0.020924513549760219 -0.0037412800759900403 0.010432097914051745 0.017716569217906979 0.017273021293018758 0.010886986001758246 0.0018310718678320899 -0.0065122691275265243 -0.011759378475939258 -0.013057295684674336 -0.010990641854786024 -0.0070281841500527019 -0.002811975217901171 0.00042299683017990954 0.0021354822806999088 0.0024432362147616925 0.0018650557342877545 0.0011881646839486063]  InputProcessing=Columns as channels (frame based)
  Out : Outport
  wires:
  In/1 -> Generated Filter Block/1
  Generated Filter Block/1 -> Out/1

== system rtlsdr_book_library/Sync Tools for Analogue Comms/Costas Loop Demodulator/Lowpass Filter1 ==
  In : Inport
  Generated Filter Block : DiscreteFir  Tag=BlockMethodSubSystem  Coefficients=[0.0011881646839486063 0.0018650557342877545 0.0024432362147616925 0.0021354822806999088 0.00042299683017990954 -0.002811975217901171 -0.0070281841500527019 -0.010990641854786024 -0.013057295684674336 -0.011759378475939258 -0.0065122691275265243 0.0018310718678320899 0.010886986001758246 0.017273021293018758 0.017716569217906979 0.010432097914051745 -0.0037412800759900403 -0.020924513549760219 -0.03484310128301845 -0.038475584236764698 -0.026293991768716812 0.003623882030617088 0.048364704584590926 0.10035872397535391 0.14905800205298941 0.18368133717457233 0.19620901660625717 0.18368133717457233 0.14905800205298941 0.10035872397535391 0.048364704584590926 0.003623882030617088 -0.026293991768716812 -0.038475584236764698 -0.03484310128301845 -0.020924513549760219 -0.0037412800759900403 0.010432097914051745 0.017716569217906979 0.017273021293018758 0.010886986001758246 0.0018310718678320899 -0.0065122691275265243 -0.011759378475939258 -0.013057295684674336 -0.010990641854786024 -0.0070281841500527019 -0.002811975217901171 0.00042299683017990954 0.0021354822806999088 0.0024432362147616925 0.0018650557342877545 0.0011881646839486063]  InputProcessing=Columns as channels (frame based)
  Out : Outport
  wires:
  Generated Filter Block/1 -> Out/1
  In/1 -> Generated Filter Block/1

== system rtlsdr_book_library/Sync Tools for Analogue Comms/Costas Loop Demodulator/Reduce Output Rate ==
  in : Inport
  Clock : simulink_extras/Flip Flops/Clock  period=1/rate*2
  Delay : Delay  DelayLength=1  InitialCondition=0
  Enabled Subsystem : $bdroot/Sync Tools for Analogue Comms/Phase Locked Loop Demodulator/Reduce Output Rate/Enabled Subsystem
  XOR : Logic  Operator=XOR  IconShape=distinctive  AllPortsSameDT=off  OutDataTypeStr=boolean
  out : Outport
  wires:
  in/1 -> Enabled Subsystem/1
  Enabled Subsystem/1 -> out/1
  XOR/1 -> Enabled Subsystem/Enable
  Clock/1 -> Delay/1, XOR/1
  Delay/1 -> XOR/2

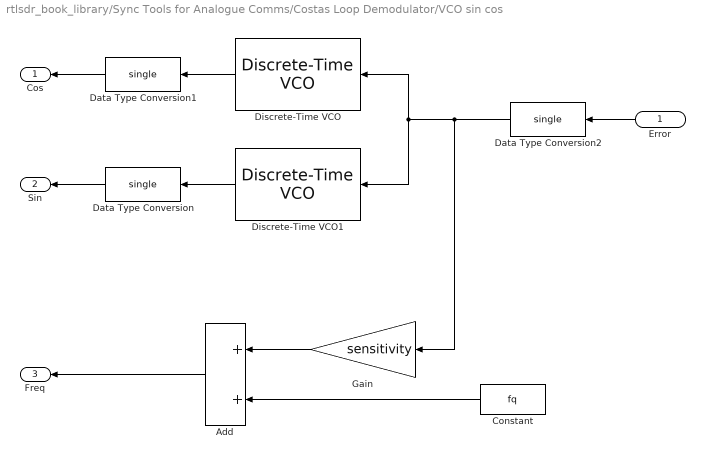
== system rtlsdr_book_library/Sync Tools for Analogue Comms/Costas Loop Demodulator/VCO sin cos ==
  Error : Inport
  Add : Sum
  Constant : Constant  Value=fq  SampleTime=1/fs
  Data Type Conversion : DataTypeConversion  OutDataTypeStr=single
  Data Type Conversion1 : DataTypeConversion  OutDataTypeStr=single
  Data Type Conversion2 : DataTypeConversion  OutDataTypeStr=single
  Discrete-Time VCO : commsynccomp2/Discrete-Time VCO  Ac=1  Fc=fq  Kc=sensitivity  Ph=pi/2  ts=1/fs
      settings: SourceProductName=Communications System Toolbox  SourceProductBaseCode=CM
  Discrete-Time VCO1 : commsynccomp2/Discrete-Time VCO  Ac=1  Fc=fq  Kc=sensitivity  Ph=0  ts=1/fs
      settings: SourceProductName=Communications System Toolbox  SourceProductBaseCode=CM
  Gain : Gain  Gain=sensitivity
  Cos : Outport
  Sin : Outport  Port=2
  Freq : Outport  Port=3
  wires:
  Data Type Conversion1/1 -> Cos/1
  Data Type Conversion/1 -> Sin/1
  Add/1 -> Freq/1
  Constant/1 -> Add/2
  Gain/1 -> Add/1
  Error/1 -> Data Type Conversion2/1
  Discrete-Time VCO/1 -> Data Type Conversion1/1
  Discrete-Time VCO1/1 -> Data Type Conversion/1
  Data Type Conversion2/1 -> Discrete-Time VCO/1, Discrete-Time VCO1/1, Gain/1

== system rtlsdr_book_library/Sync Tools for Analogue Comms/Phase Locked Loop Demodulator/Loop Filter ==
  note: _______INTEGRAL PATH_______
  note: _____PROPORTIONAL PATH_____
  sig_in : Inport
  Add : Sum
  Add1 : Sum  AccumDataTypeStr=single  OutDataTypeStr=single
  Delay : Delay  DelayLength=1  InitialCondition=0.00
  Gain1 : Gain  Gain=K2  OutDataTypeStr=single
  Gain2 : Gain  Gain=K1  ParamDataTypeStr=single
  filt_out : Outport
  wires:
  Gain1/1 -> Add/1
  Gain2/1 -> Add1/1
  sig_in/1 -> Gain1/1, Gain2/1
  Add/1 -> Add1/2, Delay/1
  Delay/1 -> Add/2
  Add1/1 -> filt_out/1
